simulink model "lecture04a_ss2tf_model"  (R2018b)
settings: Solver=VariableStepAuto  StartTime=0.0  StopTime=10.0  RelTol=1e-3
values from neighbouring files (symbols this model uses):
  A = [0 1 0 ... (first row only)    [lecture04a_ss2tf.m]
  B = [0 0 ... (first row only)    [lecture04a_ss2tf.m]
  C = [0 1 0 ... (first row only)    [lecture04a_ss2tf.m]
  D = zeros(3,2)    [lecture04a_ss2tf.m]
  GV_den = [Jm*La c*La+Jm*R+Jm*Rm KT*KV+c*R+c*Rm]    [lecture04a_ss2tf.m]
  GV_num = [KT]    [lecture04a_ss2tf.m]
undefined symbols (not defined in the file or in its folder): Atilde2, Btilde2, Ctilde2, den_tilde, Dtilde2, num_tilde
settings Model: Creator=Christopher  LastModifiedBy=Christopher

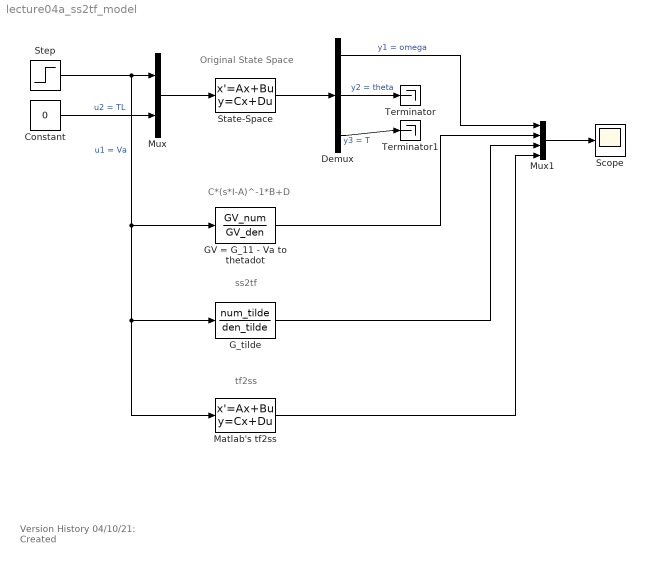
== system lecture04a_ss2tf_model ==
  note: tf2ss
  note: ss2tf
  note: C*(s*I-A)^-1*B+D
  note: Original State Space
  note: Version History
      | 04/10/21: Created
  Constant : Constant  Value=0
  Demux : Demux  Outputs=3
  GV = G_11 - Va to thetadot : TransferFcn  Numerator=GV_num  Denominator=GV_den
  G_tilde : TransferFcn  Numerator=num_tilde  Denominator=den_tilde
  Matlab's tf2ss : StateSpace  A=Atilde2  B=Btilde2  C=Ctilde2  D=Dtilde2  InitialCondition=0
  Mux : Mux  Inputs=2
  Mux1 : Mux
  Scope : Scope
  State-Space : StateSpace  A=A  B=B  C=C  D=D  InitialCondition=0
  Step : Step  SampleTime=0
  Terminator : Terminator
  Terminator1 : Terminator
  wires:
  Mux/1 -> State-Space/1
  Step/1 -> Matlab's tf2ss/1, G_tilde/1, GV = G_11 - Va to thetadot/1, Mux/1  "u1 = Va"
  Constant/1 -> Mux/2  "u2 = TL"
  State-Space/1 -> Demux/1
  Demux/2 -> Terminator/1  "y2 = theta"
  Mux1/1 -> Scope/1
  Demux/1 -> Mux1/1  "y1 = omega"
  Demux/3 -> Terminator1/1  "y3 = T"
  GV = G_11 - Va to thetadot/1 -> Mux1/2
  G_tilde/1 -> Mux1/3
  Matlab's tf2ss/1 -> Mux1/4
